simulink model "Practica1"  (R2024a)
settings: Solver=VariableStepAuto  StartTime=0.0  StopTime=10.0  RelTol=1e-3
InitFcn:
  | m1=0.2;
  | m2=0.1;
  | l1=0.3;
  | l2=0.25;
  | g=9.81;
settings Model: Creator=ximen  LastModifiedBy=ximen

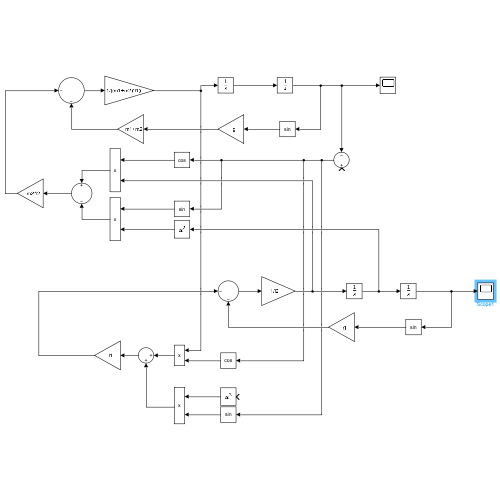
[thumbnail: Simulink's stored preview of the top-level diagram]
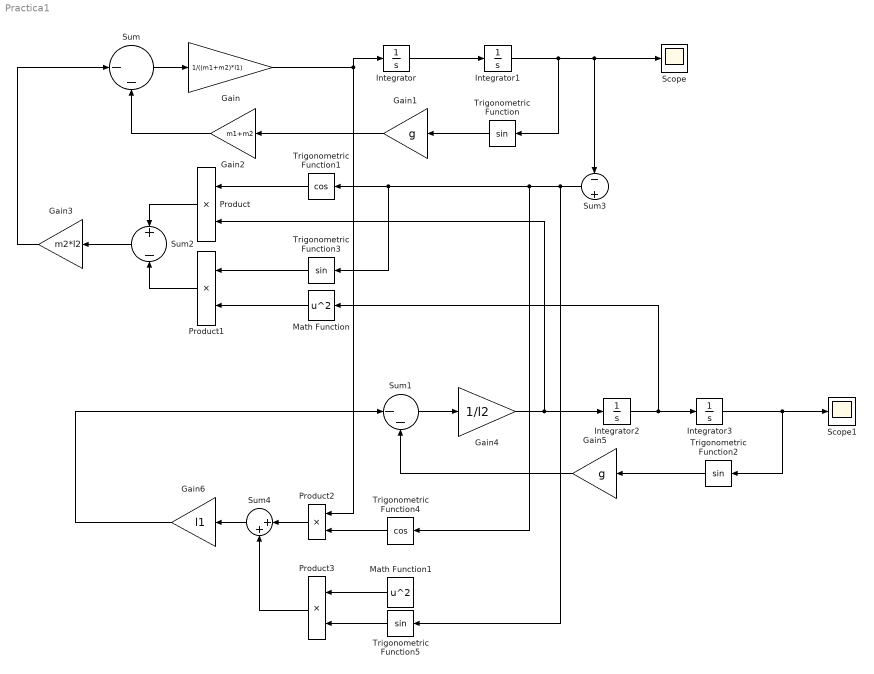
== system Practica1 ==
  Gain : Gain  Gain=1/((m1+m2)*l1)
  Gain1 : Gain  Gain=g
  Gain2 : Gain  Gain=m1+m2
  Gain3 : Gain  Gain=m2*l2
  Gain4 : Gain  Gain=1/l2
  Gain5 : Gain  Gain=g
  Gain6 : Gain  Gain=l1
  Integrator : Integrator
  Integrator1 : Integrator
  Integrator2 : Integrator
  Integrator3 : Integrator  InitialCondition=(35*pi)/180
  Math Function : Math  Operator=square
  Math Function1 : Math  Operator=square
  Product{,1..3} (4 alike) : Product
  Scope : Scope
  Scope1 : Scope
  Sum : Sum  Inputs=|--
  Sum1 : Sum  Inputs=|--
  Sum2 : Sum  Inputs=+-
  Sum3 : Sum  Inputs=-+
  Sum4 : Sum  Inputs=|++
  Trigonometric Function{,2..3,5} (4 alike) : Trigonometry
  Trigonometric Function1 : Trigonometry  Operator=cos
  Trigonometric Function4 : Trigonometry  Operator=cos
  wires:
  Sum/1 -> Gain/1
  Integrator/1 -> Integrator1/1
  Gain/1 -> Integrator/1, Product2/1
  Integrator1/1 -> Sum3/1, Scope/1, Trigonometric Function/1
  Trigonometric Function/1 -> Gain1/1
  Gain1/1 -> Gain2/1
  Gain2/1 -> Sum/2
  Integrator3/1 -> Trigonometric Function2/1, Scope1/1
  Integrator2/1 -> Math Function/1, Integrator3/1
  Gain4/1 -> Product/2, Integrator2/1
  Trigonometric Function2/1 -> Gain5/1
  Sum1/1 -> Gain4/1
  Gain5/1 -> Sum1/2
  Gain3/1 -> Sum/1
  Trigonometric Function1/1 -> Product/1
  Gain6/1 -> Sum1/1
  Trigonometric Function3/1 -> Product1/1
  Sum2/1 -> Gain3/1
  Product/1 -> Sum2/1
  Math Function/1 -> Product1/2
  Product1/1 -> Sum2/2
  Sum3/1 -> Trigonometric Function5/1, Trigonometric Function4/1, Trigonometric Function3/1, Trigonometric Function1/1
  Sum4/1 -> Gain6/1
  Product2/1 -> Sum4/1
  Trigonometric Function4/1 -> Product2/2
  Product3/1 -> Sum4/2
  Math Function1/1 -> Product3/1
  Trigonometric Function5/1 -> Product3/2
